simulink subsystem "PvtSubSys_PLAN_AP"  (R2020b)
settings: Solver=VariableStepAuto  StartTime=0.0  StopTime=10.0  RelTol=1e-3
undefined symbols (not defined in the file or in its folder): C_LongCtrl_0_Single, C_LongCtrl_0_Uint8, C_LongCtrl_Mph2Kph, magnitude, P_LongCtrl_accelTargAbsThrd, P_LongCtrl_AddVelAccelChange, P_LongCtrl_AddVelAccelThrd, P_LongCtrl_AddVelDistDesThrd, P_LongCtrl_AddVelEnable, P_LongCtrl_AddVelRefMsThrd, P_LongCtrl_ALaLowerChar, P_LongCtrl_ALaUpperCharEco, P_LongCtrl_ALaUpperCharNormal, P_LongCtrl_ALaUpperCharSport, P_LongCtrl_ALCAccLimitByDangerXAxis, P_LongCtrl_ALCAccLimitByDangerYAxis, P_LongCtrl_ALvAcceleLowerChar, P_LongCtrl_ALvAcceleUpperCharEco, P_LongCtrl_ALvAcceleUpperCharNormal, P_LongCtrl_ALvAcceleUpperCharSport, P_LongCtrl_CCaccelCCNeg2PosJerk, P_LongCtrl_CCaccelCCPosJerk, P_LongCtrl_CCaccelLowerIsLaneChange, P_LongCtrl_CCaccelMaxLCActive, P_LongCtrl_CCaccelMinECOAL, P_LongCtrl_CCaccelMinFastDecel, P_LongCtrl_CCaccelMinNoFastDecel, P_LongCtrl_CCaccelMinNormAL, P_LongCtrl_CCaccelMinSportAL, P_LongCtrl_CCaccelUpperCC, P_LongCtrl_CCaccelUpperCCSafeStop, P_LongCtrl_CCaMinNegAcceleLowerBand, P_LongCtrl_CCaMinNegAcceleUpperBand, P_LongCtrl_CCaMinPosAcceleLowerBand, P_LongCtrl_CCaMinPosAcceleUpperBand, P_LongCtrl_CCbECO, P_LongCtrl_CCbNorm, P_LongCtrl_CCbSport, P_LongCtrl_CCcoefESPSpd2IPSpd1, P_LongCtrl_CCcoefESPSpd2IPSpd2, P_LongCtrl_CCdecelCCJerk, P_LongCtrl_CCdecelCCJerkNegVLCInternalAcc, P_LongCtrl_CCfacNegAcceleLowerBand, P_LongCtrl_CCfacNegAcceleUpperBand, P_LongCtrl_CCfacPosAcceleLowerBand, P_LongCtrl_CCfacPosAcceleUpperBand, P_LongCtrl_CCkECO, P_LongCtrl_CCkNorm, P_LongCtrl_CCkSport, P_LongCtrl_CCLCIncSetSpdAdd, P_LongCtrl_CCLCIncSetSpdAddCntStartValue, P_LongCtrl_CCResumeDelayDeltaVel, P_LongCtrl_CCtAcceleTimeNeg, P_LongCtrl_CCtAcceleTimeNegCorrXAxis, P_LongCtrl_CCtAcceleTimeNegCorrYAxis, P_LongCtrl_CCtAcceleTimePos, P_LongCtrl_CCtAcceleTimePosCorrXAxis, P_LongCtrl_CCtAcceleTimePosCorrYAxis, P_LongCtrl_CCtStepVelPlan, P_LongCtrl_CCtTotVelPlan ... (+150)
libraries: simulink x62, TrueDurationTime x1
(part 3 of 7)

== system PvtSubSys_PLAN_AP/AP/AP/CCCtrl/accelCCJerkSelect ==
  VlcInternalAccK1 : Inport
  Compare To Constant : simulink/Logic and Bit Operations/Compare To Constant  relop=<  const=0  OutDataTypeStr=boolean
  Compare To Constant1 : simulink/Logic and Bit Operations/Compare To Constant  relop=>  const=0  OutDataTypeStr=boolean
  P_LongCtrl_CCaccelCCNeg2PosJerk : Constant  Value=P_LongCtrl_CCaccelCCNeg2PosJerk  OutDataTypeStr=single
  P_LongCtrl_CCaccelCCPosJerk : Constant  Value=P_LongCtrl_CCaccelCCPosJerk  OutDataTypeStr=single
  P_LongCtrl_CCdecelCCJerk : Constant  Value=P_LongCtrl_CCdecelCCJerk  OutDataTypeStr=single
  P_LongCtrl_CCdecelCCJerkNegVLCInternalAcc : Constant  Value=P_LongCtrl_CCdecelCCJerkNegVLCInternalAcc  OutDataTypeStr=single
  Switch : Switch  Criteria=u2 > Threshold
  Switch1 : Switch  Criteria=u2 > Threshold
  accelCCJerk : Outport
  decelCCJerk : Outport  Port=2
  wires:
  P_LongCtrl_CCdecelCCJerk/1 -> Switch1/1
  P_LongCtrl_CCdecelCCJerkNegVLCInternalAcc/1 -> Switch1/3  "decelCCJerk"
  Compare To Constant1/1 -> Switch1/2
  Switch1/1 -> decelCCJerk/1  "decelCCJerk"
  Switch/1 -> accelCCJerk/1  "accelCCJerk"
  P_LongCtrl_CCaccelCCPosJerk/1 -> Switch/3
  Compare To Constant/1 -> Switch/2
  VlcInternalAccK1/1 -> Compare To Constant/1, Compare To Constant1/1  "VlcInternalAccK1"
  P_LongCtrl_CCaccelCCNeg2PosJerk/1 -> Switch/1

== system PvtSubSys_PLAN_AP/AP/AP/CCCtrl/accelJerkCalc ==
  accelCCLim : Inport
  VlcInternalAcc : Inport  Port=2
  accelCCJerk : Inport  Port=3
  decelCCJerk : Inport  Port=4
  tCycle : Inport  Port=5
  Add : Sum
  Add1 : Sum
  MinMax : MinMax  Inputs=2
  MinMax1 : MinMax  Function=max  Inputs=2
  Product : Product
  Product1 : Product
  VlcInternalAcc1 : InportShadow  Port=2
  acceleratejerk1 : Constant  Value=4  OutDataTypeStr=single
  deceleratejerk1 : Constant  Value=-4  OutDataTypeStr=single
  accelCCDes : Outport
  upperJerkCC : Outport  Port=2
  lowerJerkCC : Outport  Port=3
  wires:
  acceleratejerk1/1 -> upperJerkCC/1  "upperJerkCC"
  deceleratejerk1/1 -> lowerJerkCC/1  "lowerJerkCC"
  MinMax1/1 -> accelCCDes/1  "accelCCDes"
  Add1/1 -> MinMax1/2
  Product1/1 -> Add1/2
  VlcInternalAcc1/1 -> Add1/1  "VlcInternalAcc"
  decelCCJerk/1 -> Product1/1
  tCycle/1 -> Product/2, Product1/2
  MinMax/1 -> MinMax1/1
  Add/1 -> MinMax/2
  Product/1 -> Add/2
  accelCCJerk/1 -> Product/1
  VlcInternalAcc/1 -> Add/1  "VlcInternalAcc"
  accelCCLim/1 -> MinMax/1

== system PvtSubSys_PLAN_AP/AP/AP/CCCtrl/velPlanCC ==
  VlcInternalAccK1 : Inport  OutDataTypeStr=single
  accelCCLim : Inport  Port=2
  fastDecel : Inport  Port=3
  DrivingMode : Inport  Port=4
  velSubj : Inport  Port=5  OutDataTypeStr=single
  Chart : Stateflow chart  TreatAsAtomicUnit=on
  Constant : Constant  Value=P_LongCtrl_CCdecelCCJerkNegVLCInternalAcc
  Constant1 : Constant  Value=P_LongCtrl_CCdecelCCJerk
  Constant10 : Constant  Value=P_LongCtrl_CCaccelMinNormAL  OutDataTypeStr=single
  Constant11 : Constant  Value=P_LongCtrl_CCbNorm  OutDataTypeStr=single
  Constant12 : Constant  Value=P_LongCtrl_CCkECO  OutDataTypeStr=single
  Constant13 : Constant  Value=P_LongCtrl_CCbSport  OutDataTypeStr=single
  Constant14 : Constant  Value=P_LongCtrl_CCkNorm  OutDataTypeStr=single
  Constant15 : Constant  Value=P_LongCtrl_CCbECO  OutDataTypeStr=single
  Constant16 : Constant  Value=P_LongCtrl_CCkSport  OutDataTypeStr=single
  Constant2 : Constant  Value=P_LongCtrl_CCaccelMinNoFastDecel
  Constant3 : Constant  Value=P_LongCtrl_CCaccelMinFastDecel
  Constant4 : Constant  Value=P_LongCtrl_CCtTotVelPlan  OutDataTypeStr=single
  Constant5 : Constant  Value=P_LongCtrl_CCtStepVelPlan  OutDataTypeStr=single
  Constant6 : Constant  Value=P_LongCtrl_CCaccelCCNeg2PosJerk  OutDataTypeStr=single
  Constant7 : Constant  Value=P_LongCtrl_CCaccelCCPosJerk  OutDataTypeStr=single
  Constant8 : Constant  Value=P_LongCtrl_CCaccelMinECOAL  OutDataTypeStr=single
  Constant9 : Constant  Value=P_LongCtrl_CCaccelMinSportAL  OutDataTypeStr=single
  velSubjPlanCC2ALC : Outport
  wires:
  DrivingMode/1 -> Chart/1(drivingMode)  "DrivingMode"
  velSubj/1 -> Chart/2(velSubj)  "velSubj"
  fastDecel/1 -> Chart/3(fastDecel)  "fastDecel"
  accelCCLim/1 -> Chart/4(accelCCLim)  "accelCCLim"
  VlcInternalAccK1/1 -> Chart/5(VLCInternalAccK1)  "VlcInternalAcc"
  Constant/1 -> Chart/6(P_LongCtrl_CCdecelCCJerkNegVLCInternalAcc)
  Constant1/1 -> Chart/7(P_LongCtrl_CCdecelCCJerk)
  Constant2/1 -> Chart/8(P_LongCtrl_CCaccelMinNoFastDecel)
  Constant3/1 -> Chart/9(P_LongCtrl_CCaccelMinFastDecel)
  Constant4/1 -> Chart/10(P_LongCtrl_CCtTotVelPlan)
  Constant5/1 -> Chart/11(P_LongCtrl_CCtStepVelPlan)
  Constant6/1 -> Chart/12(P_LongCtrl_CCaccelCCNeg2PosJerk)
  Constant7/1 -> Chart/13(P_LongCtrl_CCaccelCCPosJerk)
  Constant8/1 -> Chart/14(P_LongCtrl_CCaccelMinECOAL)
  Constant9/1 -> Chart/15(P_LongCtrl_CCaccelMinSportAL)
  Constant10/1 -> Chart/16(P_LongCtrl_CCaccelMinNormAL)
  Constant11/1 -> Chart/17(P_LongCtrl_CCbNorm)
  Constant14/1 -> Chart/18(P_LongCtrl_CCkNorm)
  Constant15/1 -> Chart/19(P_LongCtrl_CCbECO)
  Constant12/1 -> Chart/20(P_LongCtrl_CCkECO)
  Constant13/1 -> Chart/21(P_LongCtrl_CCbSport)
  Constant16/1 -> Chart/22(P_LongCtrl_CCkSport)
  Chart/1(velSubjPlanCC2ALC) -> velSubjPlanCC2ALC/1

== system PvtSubSys_PLAN_AP/AP/AP/FollowCtrl/AccelSupression ==
  accelFollow : Inport
  accelSubjPlanOpt : Inport  Port=2
  accelTargAbsEnable : Inport  Port=3
  velSubj : Inport  Port=4
  velTargRel : Inport  Port=5
  IDP0 : Inport  Port=6
  distTargRel : Inport  Port=7
  dangerLevel : Inport  Port=8
  laneChangeEnable : Inport  Port=9
  1-D Lookup Table : Lookup_n-D  NumberOfTableDimensions=1  BreakpointsForDimension1=P_LongCtrl_ALCAccLimitByDangerXAxis  Table=P_LongCtrl_ALCAccLimitByDangerYAxis  InternalRulePriority=Speed  RndMeth=Simplest  InputSameDT=on
  AccelSupression : Stateflow chart  TreatAsAtomicUnit=on
      settings: PortSchema="{\"entries\":[{\"content\":{\"sides\":[{\"content\":{\"connectorIds\":[\"In10\",\"In1\",\"In2\",\"In3\",\"In4\",\"In5\",\"In6\",\"In7\",\"In8\",\"In9\"]},\"type\":\"ConnectorPlacement.EquallySpacedRectSide\",\"uuid\":\"9300e1f1-bb95-41d4-adae-c883a64c9aa1\"},{\"content\":{\"connectorIds\":[\"Out1\",\"Out2\",\"Out3\"],\"side\":\"RIGHT\"},\"type\":\"ConnectorPlacement.EquallySpacedRectSide\",\"uuid\":\"008efea5-f081-441f-b580-11e25a33f47d\"},{\"content\":{\"connectorIds\":[],\"side\":\"TOP\"},\"type\":\"ConnectorPlacement.EquallySpacedRectSide\",\"uuid\":\"fa3bfdb5-3624-441a-b6df-0080d7c49dd2\"},{\"content\":{\"connectorIds\":[],\"side\":\"HIDDEN\"},\"type\":\"ConnectorPlacement.EquallySpacedRectSide\",\"uuid\":\"07e1617e-6ebd-494d-b9df-12fef96acb1d\"}]},\"type\":\"ConnectorPlacement.EquallySpacedConnector\",\"uuid\":\"901f3200-aee3-4515-88aa-e0e7a99820ae\"}],\"packageUris\":[\"http://schema.mathworks.com/mf0/Connector/R2020b\"],\"version\":\"1.0\"}"
  Constant : Constant  Value=P_LongCtrl_DangerLevelEnterThrd  OutDataTypeStr=single
  Constant2 : Constant  Value=P_LongCtrl_FollowaccelMinAccelSupressionEnter
  Constant3 : Constant  Value=P_LongCtrl_FollowaccelMinAccelSupressionExit
  Constant4 : Constant  Value=P_LongCtrl_DangerLevelExitThrd  OutDataTypeStr=single
  DecelJudge : MATLAB Function  TreatAsAtomicUnit=on
  MinMax : MinMax  Function=max  Inputs=2
  Signal Copy : SignalConversion  OverrideOpt=off
  Signal Copy1 : SignalConversion  OverrideOpt=off
  Switch : Switch  Criteria=u2 > Threshold
  Terminator : Terminator
  Terminator1 : Terminator
  accelFollowAfterLaneChangeSupress : Outport
  tStartDecel : Outport  Port=2
  wires:
  Signal Copy/1 -> AccelSupression/4(laneChangeEnable)  "LongCtrl_laneChangeEnable"
  Signal Copy1/1 -> AccelSupression/10(dangerLevel)  "LongCtrl_dangerLevel"
  dangerLevel/1 -> Signal Copy1/1, 1-D Lookup Table/1
  [accelFollow] -> MinMax/2
  MinMax/1 -> Switch/1
  Constant/1 -> AccelSupression/8(P_LongCtrl_DangerLevelEnterThrd)
  Constant4/1 -> AccelSupression/9(P_LongCtrl_DangerLevelExitThrd)
  accelTargAbsEnable/1 -> AccelSupression/2(accelTargAbsEnable)
  velSubj/1 -> AccelSupression/3(velSubj)
  velTargRel/1 -> AccelSupression/1(velTargRel)
  laneChangeEnable/1 -> Signal Copy/1
  accelSubjPlanOpt/1 -> DecelJudge/1(accelSubjPlanOpt)  "accelSubjPlanOpt"
  AccelSupression/1(accelSupressionEnable) -> Switch/2  "LongCtrl_accelSupressionEnable"
  1-D Lookup Table/1 -> MinMax/1  "LongCtrl_AccelSupreReq"
  accelFollow/1 -> Switch/3, [accelFollow]
  Switch/1 -> accelFollowAfterLaneChangeSupress/1  "LongCtrl_accelFollowAfterLaneChangeSupress"
  DecelJudge/1(tStartDecel) -> tStartDecel/1  "LongCtrl_tStartDecel"
  IDP0/1 -> DecelJudge/2(IDP0)  "IDP0"
  AccelSupression/2(distAccelSupressionMinEnter) -> Terminator/1  "LongCtrl_distAccelSupressionEnter"
  distTargRel/1 -> AccelSupression/5(distTargRel)
  Constant2/1 -> AccelSupression/6(P_LongCtrl_FollowaccelMinAccelSupressionEnter)
  Constant3/1 -> AccelSupression/7(P_LongCtrl_FollowaccelMinAccelSupressionExit)
  AccelSupression/3(distAccelSupressionMinExit) -> Terminator1/1  "LongCtrl_distAccelSupressionExit"

== system PvtSubSys_PLAN_AP/AP/AP/FollowCtrl/AccelTargAbsEnableJudge ==
  accelTargAbsFilt : Inport
  distTargRel : Inport  Port=2
  tCycle : Inport  Port=3
  IDP0 : Inport  Port=4  OutDataTypeStr=uint8
  AccelTargAbsEnableJudge : Stateflow chart  TreatAsAtomicUnit=on
  P_LongCtrl_FollowaccelTargAbsEnableNegJerk : Constant  Value=P_LongCtrl_FollowaccelTargAbsEnableNegJerk  OutDataTypeStr=single
  P_LongCtrl_FollowaccelTargAbsEnableNegMax : Constant  Value=P_LongCtrl_FollowaccelTargAbsEnableNegMax  OutDataTypeStr=single
  P_LongCtrl_FollowaccelTargAbsEnablePosJerk : Constant  Value=P_LongCtrl_FollowaccelTargAbsEnablePosJerk  OutDataTypeStr=single
  P_LongCtrl_FollowaccelTargAbsEnableRangeMax : Constant  Value=P_LongCtrl_FollowaccelTargAbsEnableRangeMax  OutDataTypeStr=single
  P_LongCtrl_FollowaccelTargAbsExitNegMin : Constant  Value=P_LongCtrl_FollowaccelTargAbsExitNegMin  OutDataTypeStr=single
  P_LongCtrl_FollowdistTargRelEnableAccelTargAbsThres : Constant  Value=P_LongCtrl_FollowdistTargRelEnableAccelTargAbsThres  OutDataTypeStr=single
  Tapped Delay : simulink/Discrete/Tapped Delay  vinit=0.0  samptime=-1  NumDelays=1  DelayOrder=Newest  includeCurrent=on
  accelTargAbsEnable : Outport
  wires:
  distTargRel/1 -> AccelTargAbsEnableJudge/2(distTargRel)
  tCycle/1 -> AccelTargAbsEnableJudge/4(tCycle)
  P_LongCtrl_FollowaccelTargAbsExitNegMin/1 -> AccelTargAbsEnableJudge/7(C_accelTargAbsExitNegMin)
  P_LongCtrl_FollowaccelTargAbsEnableRangeMax/1 -> AccelTargAbsEnableJudge/10(C_accelTargAbsEnableRangeMax)
  P_LongCtrl_FollowaccelTargAbsEnablePosJerk/1 -> AccelTargAbsEnableJudge/8(C_accelTargAbsEnablePosJerk)
  P_LongCtrl_FollowaccelTargAbsEnableNegMax/1 -> AccelTargAbsEnableJudge/5(C_accelTargAbsEnableNegMax)
  accelTargAbsFilt/1 -> AccelTargAbsEnableJudge/3(accelTargAbsFilt)
  P_LongCtrl_FollowdistTargRelEnableAccelTargAbsThres/1 -> AccelTargAbsEnableJudge/9(C_distTargRelEnableAccelTargAbsThres)
  P_LongCtrl_FollowaccelTargAbsEnableNegJerk/1 -> AccelTargAbsEnableJudge/6(C_accelTargAbsEnableNegJerk)
  AccelTargAbsEnableJudge/1(accelTargAbs) -> accelTargAbsEnable/1
  IDP0/1 -> Tapped Delay/1  "IDP0"
  Tapped Delay/1 -> AccelTargAbsEnableJudge/1(IDP0)

== system PvtSubSys_PLAN_AP/AP/AP/FollowCtrl/AccelTargFilter ==
  IDP0 : Inport  OutDataTypeStr=uint8
  IDP2 : Inport  Port=2  OutDataTypeStr=uint8
  IDP3 : Inport  Port=3  OutDataTypeStr=uint8
  accelTargAbsP0 : Inport  Port=4
  accelTargAbsP2 : Inport  Port=5
  accelTargAbsP3 : Inport  Port=6
  Tapped Delay : simulink/Discrete/Tapped Delay  vinit=0.0  samptime=-1  NumDelays=1  DelayOrder=Newest  includeCurrent=on
  Tapped Delay1 : simulink/Discrete/Tapped Delay  vinit=0.0  samptime=-1  NumDelays=1  DelayOrder=Newest  includeCurrent=on
  Tapped Delay2 : simulink/Discrete/Tapped Delay  vinit=0.0  samptime=-1  NumDelays=1  DelayOrder=Newest  includeCurrent=on
  accelTargAbsFilter : Stateflow chart  TreatAsAtomicUnit=on
  accelTargAbsFilt : Outport
  wires:
  Tapped Delay2/1 -> accelTargAbsFilter/3(IDP3)
  Tapped Delay1/1 -> accelTargAbsFilter/2(IDP2)
  Tapped Delay/1 -> accelTargAbsFilter/1(IDP0)
  accelTargAbsP3/1 -> accelTargAbsFilter/6(accelTargAbsP3)
  accelTargAbsP2/1 -> accelTargAbsFilter/5(accelTargAbsP2)
  IDP3/1 -> Tapped Delay2/1
  IDP2/1 -> Tapped Delay1/1
  IDP0/1 -> Tapped Delay/1  "IDP0"
  accelTargAbsP0/1 -> accelTargAbsFilter/4(accelTargAbsP0)
  accelTargAbsFilter/1(accelTargAbsFiltP0) -> accelTargAbsFilt/1  "accelTargAbsFilt"

== system PvtSubSys_PLAN_AP/AP/AP/FollowCtrl/DecelToStopCtrl ==
  accelFollow : Inport
  distDesCur : Inport  Port=2
  velTargAbs : Inport  Port=3
  accelTargAbsFilt : Inport  Port=4
  distTargRel : Inport  Port=5
  velSubj : Inport  Port=6
  ACCModeSts : Inport  Port=7  OutDataTypeStr=uint8
  DrvOFF_Req : Inport  Port=8
  axvRoadSlopeMs2 : Inport  Port=9
  ObjMovingStateP0 : Inport  Port=10
  DecelToStopCtrl : Subsystem
  accelFollowAfterDecelToStop : Outport
  ForceStop : Outport  Port=2
  wires:
  ObjMovingStateP0/1 -> DecelToStopCtrl/10(ObjMovingStateP0)
  DrvOFF_Req/1 -> DecelToStopCtrl/8(DrvOFF_Req)
  velTargAbs/1 -> DecelToStopCtrl/6(velTargAbs)
  ACCModeSts/1 -> DecelToStopCtrl/7(ACCModeSts)
  distDesCur/1 -> DecelToStopCtrl/5(distDesCur)
  DecelToStopCtrl/1(FollowAccel) -> accelFollowAfterDecelToStop/1  "LongCtrl_accelFollowAfterDecelToStop"
  accelTargAbsFilt/1 -> DecelToStopCtrl/2(accelTargAbs)
  distTargRel/1 -> DecelToStopCtrl/3(distTargRel)
  velSubj/1 -> DecelToStopCtrl/4(velSubj)
  accelFollow/1 -> DecelToStopCtrl/1(FollowAccelMPC)  "accelFollwBeforeDecelToStop"
  axvRoadSlopeMs2/1 -> DecelToStopCtrl/9(axvRoadSlopeMs2)
  DecelToStopCtrl/2(ForceStop) -> ForceStop/1  "LongCtrl_ForceStop"

== system PvtSubSys_PLAN_AP/AP/AP/FollowCtrl/DistDesCalc ==
  velTargAbsPlanTerminate : Inport
  timeGap : Inport  Port=2
  distTargRel : Inport  Port=3
  velTargRel : Inport  Port=4
  velSubj : Inport  Port=5
  1-D Lookup Table : Lookup_n-D  NumberOfTableDimensions=1  BreakpointsForDimension1=P_LongCtrl_FollowdistDesCompensionXAxis  Table=P_LongCtrl_FollowdistDesCompensionYAxis  ExtrapMethod=Clip  InternalRulePriority=Speed  RndMeth=Simplest  InputSameDT=on
  Constant36 : Constant  Value=P_LongCtrl_FollowDistDesCompensionVelRelThresMin  OutDataTypeStr=single
  Constant37 : Constant  Value=P_LongCtrl_FollowDistDesCompensionVelRelThresMax  OutDataTypeStr=single
  DesireDistance1 : Lookup_n-D  BreakpointsForDimension1=[1,2,3,4]  BreakpointsForDimension2=P_LongCtrl_FollowdistDesX2Axis  BreakpointsForDimension1DataTypeStr=single  BreakpointsForDimension2DataTypeStr=single  Table=P_LongCtrl_FollowdistDesYAxis  TableDataTypeStr=single  ExtrapMethod=Clip  OutDataTypeStr=single  RndMeth=Simplest
      settings: InputPortMap=u0,u1
  DesireDistance2 : Lookup_n-D  BreakpointsForDimension1=[1,2,3,4]  BreakpointsForDimension2=P_LongCtrl_FollowdistDesX2Axis  BreakpointsForDimension1DataTypeStr=single  BreakpointsForDimension2DataTypeStr=single  Table=P_LongCtrl_FollowdistDesYAxis  TableDataTypeStr=single  ExtrapMethod=Clip  OutDataTypeStr=single  RndMeth=Simplest
      settings: InputPortMap=u0,u1
  DesireDistance3 : Lookup_n-D  BreakpointsForDimension1=[1,2,3,4]  BreakpointsForDimension2=P_LongCtrl_FollowdistDesX2Axis  BreakpointsForDimension1DataTypeStr=single  BreakpointsForDimension2DataTypeStr=single  Table=P_LongCtrl_FollowdistDesYAxis  TableDataTypeStr=single  ExtrapMethod=Clip  OutDataTypeStr=single  RndMeth=Simplest
      settings: InputPortMap=u0,u1
  Gain9 : Gain  Gain=3.6
  Lookup Table Dynamic : simulink/Lookup Tables/Lookup Table Dynamic  LookUpMeth=Interpolation-Use End Values  OutDataType=fixdt('single')  OutScaling=[]  OutputDataTypeScalingMode=Specify via dialog  OutDataTypeStr=single  DoSatur=off
  Matrix Concatenate1 : Concatenate
  Matrix Concatenate2 : Concatenate
  Min : MinMax  Inputs=2
  Subtract1 : Sum
  Subtract2 : Sum  Inputs=-+
  Subtract5 : Sum
  distDesPlanCorr : Outport
  distDesCur : Outport  Port=2
  wires:
  Subtract2/1 -> Matrix Concatenate2/1
  DesireDistance2/1 -> distDesCur/1
  [timeGap] -> DesireDistance2/1
  velSubj/1 -> Subtract1/2, DesireDistance2/2, 1-D Lookup Table/1
  [distTargRel] -> Subtract2/1
  DesireDistance1/1 -> Subtract2/2
  Subtract1/1 -> DesireDistance1/2
  [timeGap] -> DesireDistance1/1
  Min/1 -> distDesPlanCorr/1
  Subtract5/1 -> Min/2
  distTargRel/1 -> [distTargRel], Subtract5/1
  Lookup Table Dynamic/1 -> Subtract5/2
  Matrix Concatenate2/1 -> Lookup Table Dynamic/3
  Constant36/1 -> Matrix Concatenate1/1
  Gain9/1 -> Lookup Table Dynamic/1
  1-D Lookup Table/1 -> Matrix Concatenate2/2
  Constant37/1 -> Matrix Concatenate1/2
  Matrix Concatenate1/1 -> Lookup Table Dynamic/2
  velTargRel/1 -> Subtract1/1, Gain9/1
  velTargAbsPlanTerminate/1 -> DesireDistance3/2
  DesireDistance3/1 -> Min/1  "LongCtrl_distDesPlan"
  timeGap/1 -> [timeGap], DesireDistance3/1

== system PvtSubSys_PLAN_AP/AP/AP/FollowCtrl/DistRelPlanTerminateCalc ==
  accelTargAbsEnable : Inport
  velTargAbs : Inport  Port=2
  velTargAbsPlanTerminate : Inport  Port=3
  distDesPlanCorr : Inport  Port=4
  distTargRel : Inport  Port=5
  velSubj : Inport  Port=6
  1-D Lookup Table : Lookup_n-D  NumberOfTableDimensions=1  BreakpointsForDimension1=[0 2]  Table=[0 2]  ExtrapMethod=Clip  InternalRulePriority=Speed  RndMeth=Simplest  InputSameDT=on
  DistRelPlanTerminateCalc2 : MATLAB Function  TreatAsAtomicUnit=on
  distRelPlanTerminate : Outport
  tTargStop : Outport  Port=2
  distTargPlan : Outport  Port=3
  wires:
  DistRelPlanTerminateCalc2/3(distTargPlan) -> distTargPlan/1
  DistRelPlanTerminateCalc2/2(tTargStop) -> tTargStop/1
  1-D Lookup Table/1 -> DistRelPlanTerminateCalc2/6(DterminateMin)
  velSubj/1 -> DistRelPlanTerminateCalc2/7(velSubj), 1-D Lookup Table/1
  velTargAbs/1 -> DistRelPlanTerminateCalc2/4(vf)
  DistRelPlanTerminateCalc2/1(Dterminate) -> distRelPlanTerminate/1  "distRelPlanTerminate"
  velTargAbsPlanTerminate/1 -> DistRelPlanTerminateCalc2/3(velTargAbsPlanTerminate)
  distDesPlanCorr/1 -> DistRelPlanTerminateCalc2/2(distDesPlanCorr)
  distTargRel/1 -> DistRelPlanTerminateCalc2/1(R)
  accelTargAbsEnable/1 -> DistRelPlanTerminateCalc2/5(af)

== system PvtSubSys_PLAN_AP/AP/AP/FollowCtrl/FollowBandJerkCalc ==
  Gap : Inport
  accelFollow : Inport  Port=2
  PlauCheckEnable : Inport  Port=3
  ttc : Inport  Port=4
  ForceStop : Inport  Port=5
  VlcInternalAccK1 : Inport  Port=6
  distTargRel : Inport  Port=7
  velSubj : Inport  Port=8
  ACCModeSts : Inport  Port=9  OutDataTypeStr=uint8
  tCycle : Inport  Port=10
  velTargRel : Inport  Port=11
  IDP0 : Inport  Port=12
  axvRoadSlopeMs2 : Inport  Port=13
  accelTargAbsFilt : Inport  Port=14
  AccelFollowAfterJerk : Subsystem
  AccelFollowJerkCalc : Subsystem
  DecelFollowJerkCalc : Subsystem
  LP : Subsystem
  Subsystem : Subsystem
  Terminator : Terminator
  upperBandFollow : Outport
  lowerBandFollow : Outport  Port=2
  " upperJerkFollow" : Outport  Port=3
  lowerJerkFollow : Outport  Port=4
  accelFollowAfterJerk : Outport  Port=5
  wires:
  accelTargAbsFilt/1 -> DecelFollowJerkCalc/10(accelTargAbsFilt)
  PlauCheckEnable/1 -> Terminator/1
  ttc/1 -> DecelFollowJerkCalc/7(ttc)
  velTargRel/1 -> DecelFollowJerkCalc/6(velTargRel)
  Gap/1 -> DecelFollowJerkCalc/5(Gap)
  tCycle/1 -> AccelFollowAfterJerk/3(tCycle), DecelFollowJerkCalc/1(tCycle)
  distTargRel/1 -> DecelFollowJerkCalc/2(distTargRel)
  velSubj/1 -> [velSubj], DecelFollowJerkCalc/3(velSubj)
  ACCModeSts/1 -> DecelFollowJerkCalc/4(ACCModeSts)
  VlcInternalAccK1/1 -> AccelFollowAfterJerk/2(VlcInternalAccK1), AccelFollowJerkCalc/1(VlcInternalAccK1), DecelFollowJerkCalc/11(VlcInternalAccK1)
  DecelFollowJerkCalc/1(decelFollowJerk) -> lowerJerkFollow/1, AccelFollowAfterJerk/4(lowerJerkFollow)  "LongCtrl_lowerJerkFollow"
  AccelFollowJerkCalc/1(accelFollowJerk) -> " upperJerkFollow"/1, AccelFollowAfterJerk/5(" upperJerkFollow")  "LongCtrl_upperJerkFollow"
  LP/1(accelFollowFilt) -> AccelFollowJerkCalc/2(FollowAccele), Subsystem/1(accelFollowFilt), AccelFollowAfterJerk/1(accelFollow)  "accelFollow"
  AccelFollowAfterJerk/1(accelFollowAfterJerk) -> accelFollowAfterJerk/1
  Subsystem/1(upperBandFollow) -> upperBandFollow/1
  Subsystem/2(lowerBandFollow) -> lowerBandFollow/1
  accelFollow/1 -> LP/1(accelFollow)  "accelFollow"
  ForceStop/1 -> DecelFollowJerkCalc/8(ForceStop)
  IDP0/1 -> LP/2(IDP0)
  axvRoadSlopeMs2/1 -> DecelFollowJerkCalc/9(axvRoadSlopeMs2)
  [velSubj] -> AccelFollowJerkCalc/3(velSubj)

== system PvtSubSys_PLAN_AP/AP/AP/FollowCtrl/PlausibilityCheck ==
  FollowAcceleK1 : Inport
  accelSubjPlan : Inport  Port=2
  num : Inport  Port=3
  velTargAbs : Inport  Port=4
  distRelPlanTerminate : Inport  Port=5
  velSubj : Inport  Port=6
  IDP0 : Inport  Port=7
  distTargRel : Inport  Port=8
  ACCMode : Inport  Port=9
  velTargRel : Inport  Port=10
  accelTargAbsEnable : Inport  Port=11
  distDesCur : Inport  Port=12
  Bus Creator : BusCreator  Inputs=12
  Bus Selector : BusSelector  OutputSignals=accelSubjPlan,velSubj,velTargAbs,distRelPlanTerminate,num,IDP0,FollowAcceleK1,distTargRel
  Bus Selector1 : BusSelector  OutputSignals=velTargAbs,distTargRel,ACCMode
  Bus Selector2 : BusSelector  OutputSignals=velTargRel,accelTargAbsEnable,distDesCur,velSubj,distTargRel
  PlausibilityCheck : MATLAB Function  TreatAsAtomicUnit=on
  StandstillOverride : Stateflow chart  TreatAsAtomicUnit=on
  StandstillOverrideAccelLimit : Subsystem
  Subsystem : Subsystem
  Tapped Delay : simulink/Discrete/Tapped Delay  vinit=0.0  samptime=-1  NumDelays=1  DelayOrder=Newest  includeCurrent=on
  PlauCheckEnable : Outport
  followAcceleStandstillOverride : Outport  Port=2
  wires:
  Bus Selector1/3 -> StandstillOverride/4(ACCMode)  "<ACCMode>"
  Bus Selector1/1 -> StandstillOverride/2(velTargAbs)  "<velTargAbs>"
  Bus Selector1/2 -> StandstillOverride/3(distTargRel)  "<distTargRel>"
  StandstillOverrideAccelLimit/1(followAcceleStandstillOverride) -> followAcceleStandstillOverride/1  "followAcceleStandstillOverride"
  StandstillOverride/2(coefStandstillOverride) -> StandstillOverrideAccelLimit/3(coefStandstillOverride)  "LongCtrl_coefStandstillOverride"
  ACCMode/1 -> Bus Creator/9  "ACCMode"
  Bus Selector/8 -> PlausibilityCheck/8(distTargRel)  "<distTargRel>"
  Bus Selector/7 -> PlausibilityCheck/7(FollowAcceleK1)  "<FollowAcceleK1>"
  Bus Selector/6 -> Tapped Delay/1  "<IDP0>"
  Bus Selector/5 -> PlausibilityCheck/5(num)  "<num>"
  Bus Selector/4 -> PlausibilityCheck/4(distRelPlanTerminate)  "<distRelPlanTerminate>"
  Bus Selector/3 -> PlausibilityCheck/3(velTargAbs)  "<velTargAbs>"
  Bus Selector/2 -> PlausibilityCheck/2(velSubj)  "<velSubj>"
  Bus Selector/1 -> PlausibilityCheck/1(FollowAccele)  "<accelSubjPlan>"
  Bus Creator/1 -> Bus Selector2/1, Bus Selector1/1, Bus Selector/1
  distTargRel/1 -> Bus Creator/8  "distTargRel"
  FollowAcceleK1/1 -> Bus Creator/7  "FollowAcceleK1"
  IDP0/1 -> Bus Creator/6  "IDP0"
  num/1 -> Bus Creator/5  "num"
  distRelPlanTerminate/1 -> Bus Creator/4  "distRelPlanTerminate"
  velTargAbs/1 -> Bus Creator/3  "velTargAbs"
  velSubj/1 -> Bus Creator/2  "velSubj"
  accelSubjPlan/1 -> Bus Creator/1  "accelSubjPlan"
  PlausibilityCheck/2(PlauCheckEnable) -> PlauCheckEnable/1
  Tapped Delay/1 -> PlausibilityCheck/6(IDP0)
  PlausibilityCheck/1(FollowAccele_Plau) -> StandstillOverride/1(FollowAccele_Plau), StandstillOverrideAccelLimit/1(followAccel_Plau)  "LongCtrl_followAccel_Plau"
  StandstillOverride/1(standstillOverrideCondition) -> StandstillOverrideAccelLimit/2(standstillOverrideCondition)  "LongCtrl_standstillOverrideCondition"
  velTargRel/1 -> Bus Creator/10  "velTargRel"
  accelTargAbsEnable/1 -> Bus Creator/11  "accelTargAbsEnable"
  distDesCur/1 -> Bus Creator/12  "distDesCur"
  Bus Selector2/1 -> Subsystem/1(velTargRel)  "<velTargRel>"
  Bus Selector2/2 -> Subsystem/2(accelTargAbsEnable)  "<accelTargAbsEnable>"
  Bus Selector2/3 -> Subsystem/3(distDesCur)  "<distDesCur>"
  Bus Selector2/4 -> Subsystem/4(velSubj)  "<velSubj>"
  Bus Selector2/5 -> Subsystem/5(distTargRel)  "<distTargRel>"
  Subsystem/1(quickDecel) -> StandstillOverrideAccelLimit/4(quickDecel)  "LongCtrl_quickDecel"

== system PvtSubSys_PLAN_AP/AP/AP/FollowCtrl/SlopeStartupAssist ==
  accelFollowAfterLaneChangeSupress : Inport
  axvRoadSlopeMs2 : Inport  Port=2
  velSubj : Inport  Port=3
  velTargRel : Inport  Port=4
  distTargRel : Inport  Port=5
  ACCModeSts : Inport  Port=6  OutDataTypeStr=uint8
  tCycle : Inport  Port=7
  distDesCur : Inport  Port=8
  velTargAbs : Inport  Port=9
  1-D Lookup Table : Lookup_n-D  NumberOfTableDimensions=1  BreakpointsForDimension1=P_LongCtrl_FollowAccelAddSlopeAssistXAxis  Table=P_LongCtrl_FollowAccelAddSlopeAssistYAxis  ExtrapMethod=Clip  InternalRulePriority=Speed  RndMeth=Simplest  InputSameDT=on
  Add : Sum
  Chart : Stateflow chart  TreatAsAtomicUnit=on
  Chart1 : Stateflow chart  TreatAsAtomicUnit=on
  Compare To Constant : simulink/Logic and Bit Operations/Compare To Constant  relop=<=  const=2  OutDataTypeStr=boolean
  Compare To Constant1 : simulink/Logic and Bit Operations/Compare To Constant  relop=>  const=0.8  OutDataTypeStr=boolean
  Compare To Constant2 : simulink/Logic and Bit Operations/Compare To Constant  relop=<  const=0.5  OutDataTypeStr=boolean
  Compare To Constant3 : simulink/Logic and Bit Operations/Compare To Constant  relop=>  const=0.15  OutDataTypeStr=boolean
  Constant : Constant  Value=P_LongCtrl_FollowAccelSlopeAssistStep  OutDataTypeStr=single
  Logical Operator : Logic  Inputs=4  AllPortsSameDT=off  OutDataTypeStr=boolean
  Product : Product
  accelFollowSlopeAssist : Outport
  wires:
  accelFollowAfterLaneChangeSupress/1 -> Chart1/2(accelFollowAfterLaneChangeSupress), Add/1, Compare To Constant3/1, Compare To Constant2/1
  axvRoadSlopeMs2/1 -> 1-D Lookup Table/1, Compare To Constant1/1  "axvRoadSlopeMs2"
  velSubj/1 -> Chart1/1(velSubj), Compare To Constant/1  "velSubj"
  Compare To Constant2/1 -> Logical Operator/1
  Compare To Constant3/1 -> Logical Operator/2
  Compare To Constant1/1 -> Logical Operator/4
  Compare To Constant/1 -> Logical Operator/3
  Logical Operator/1 -> Chart/1(slopeStartupAssist)  "LongCtrl_slopeStartupAssist"
  1-D Lookup Table/1 -> Chart/2(accelSlopeAssistMax)
  Constant/1 -> Chart/3(accelSlopeAssistStep)
  Add/1 -> Product/1
  Chart/1(accelSlopeAssist) -> Add/2  "LongCtrl_accelFollowSlopeAssist"
  velTargAbs/1 -> Chart1/3(velTargAbs)
  distDesCur/1 -> Chart1/4(distDesCur)
  distTargRel/1 -> Chart1/5(distTargRel)
  velTargRel/1 -> Chart1/6(velTargRel)
  ACCModeSts/1 -> Chart1/7(ACCModeSts)
  tCycle/1 -> Chart1/8(tCycle)
  Chart1/1(coefVelDist2Accel) -> Product/2  "LongCtrl_coefVelDist2AccelStartUp"
  Product/1 -> accelFollowSlopeAssist/1

== system PvtSubSys_PLAN_AP/AP/AP/FollowCtrl/TTC ==
  velTargRel : Inport
  distTargRel : Inport  Port=2
  Constant : Constant  Value=0.01  OutDataTypeStr=single
  Gain : Gain  Gain=-1
  MinMax : MinMax  Function=max  Inputs=2
  Product1 : Product  Inputs=*/
  ttc : Outport
  wires:
  Gain/1 -> MinMax/1
  Constant/1 -> MinMax/2
  Product1/1 -> ttc/1
  MinMax/1 -> Product1/2
  velTargRel/1 -> Gain/1
  distTargRel/1 -> Product1/1

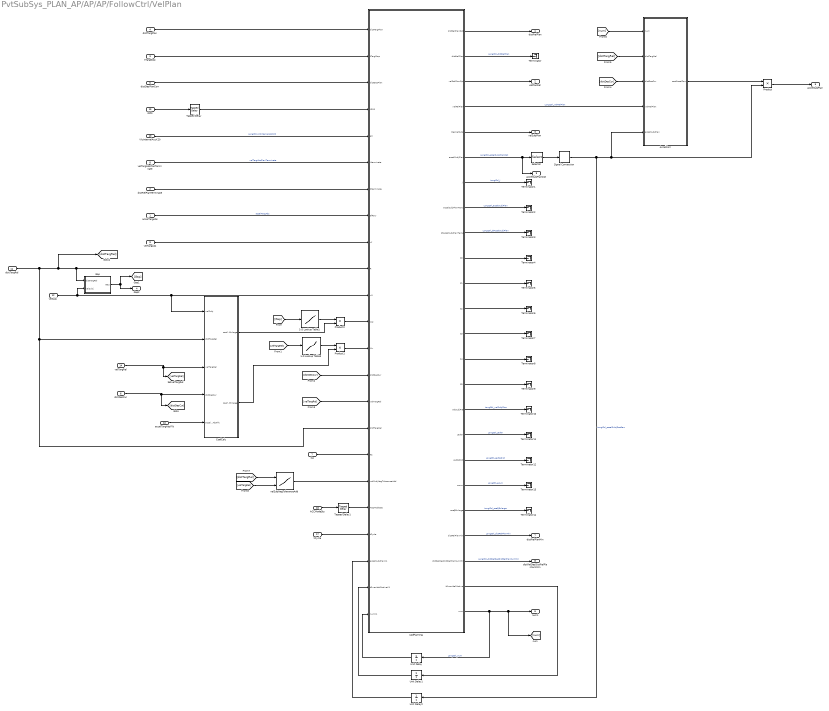
== system PvtSubSys_PLAN_AP/AP/AP/FollowCtrl/VelPlan ==
  accelTargAbs : Inport
  distRelPlanTerminate : Inport  Port=2
  tTargStop : Inport  Port=3
  distTargPlan : Inport  Port=4
  distDesPlanCorr : Inport  Port=5
  distDesCur : Inport  Port=6
  ttc : Inport  Port=7
  velTargAbsPlanTerminate : Inport  Port=8
  velTargAbs : Inport  Port=9
  accelTargAbsFilt : Inport  Port=10
  distTargRel : Inport  Port=11
  velSubj : Inport  Port=12
  VlcInternalAccK20 : Inport  Port=13
  velTargRel : Inport  Port=14
  IDP0 : Inport  Port=15  OutDataTypeStr=uint8
  ACCModeSts : Inport  Port=16  OutDataTypeStr=uint8
  tCycle : Inport  Port=17
  1-D Lookup Table1 : Lookup_n-D  NumberOfTableDimensions=1  BreakpointsForDimension1=P_LongCtrl_FollowWdCoefXAxis  Table=P_LongCtrl_FollowWdCoefYAxis  ExtrapMethod=Clip  InternalRulePriority=Speed  RndMeth=Simplest  InputSameDT=on
  1-D Lookup Table3 : Lookup_n-D  NumberOfTableDimensions=1  BreakpointsForDimension1=P_LongCtrl_FollowWvCoefXAxis  Table=P_LongCtrl_FollowWvCoefYAxis  ExtrapMethod=Clip  InternalRulePriority=Speed  RndMeth=Simplest  InputSameDT=on
  AccelCorr : MATLAB Function  TreatAsAtomicUnit=on
  CoefCalc : MATLAB Function  TreatAsAtomicUnit=on
  Gap : Subsystem
  Product : Product
  Product1 : Product
  Product2 : Product
  Selector : Selector  InputPortWidth=40  IndexOptions=Index vector (dialog)  Indices=1  OutputSizes=1
  Signal Conversion : SignalConversion  OverrideOpt=off
  Tapped Delay : simulink/Discrete/Tapped Delay  vinit=0.0  samptime=-1  NumDelays=1  DelayOrder=Newest  includeCurrent=on
  Tapped Delay1 : simulink/Discrete/Tapped Delay  vinit=0.0  samptime=-1  NumDelays=1  DelayOrder=Newest  includeCurrent=on
  Terminator{,1..14} (15 alike) : Terminator
  Unit Delay : UnitDelay  InitialCondition=2  SampleTime=-1  HasFrameUpgradeWarning=on
  Unit Delay1 : UnitDelay  SampleTime=-1  HasFrameUpgradeWarning=on
  Unit Delay2 : UnitDelay  SampleTime=-1  HasFrameUpgradeWarning=on
  spdPlanning : MATLAB Function  TreatAsAtomicUnit=on
  velSubjNegToleranceAdd : Lookup_n-D  BreakpointsForDimension1=P_LongCtrl_FollowVelSubjNegToleranceAddX1Axis  BreakpointsForDimension2=P_LongCtrl_FollowVelSubjNegToleranceAddX2Axis  Table=P_LongCtrl_FollowVelSubjNegToleranceAddYAxis  ExtrapMethod=Clip  InternalRulePriority=Speed  RndMeth=Simplest  InputSameDT=on
      settings: InputPortMap=u0,u1
  distRelPlan : Outport  OutDataTypeStr=single
  velPlanRel : Outport  Port=2  OutDataTypeStr=single
  velSubjPlan : Outport  Port=3  OutDataTypeStr=single
  Gap2 : Outport  Port=4  OutDataTypeStr=single
  accelSubjPlan : Outport  Port=5  OutDataTypeStr=single
  num1 : Outport  Port=6  OutDataTypeStr=single
  distRelPlanMin : Outport  Port=7  OutDataTypeStr=single
  distRelDesDistRelPlanNumMin : Outport  Port=8  OutDataTypeStr=single
  accelSubjPlanOpt : Outport  Port=9
  wires:
  ACCModeSts/1 -> Tapped Delay1/1
  velSubjNegToleranceAdd/1 -> spdPlanning/18(velSubjNegToleranceAdd)
  [velTargRel] -> velSubjNegToleranceAdd/2
  [distTargRel] -> velSubjNegToleranceAdd/1
  tCycle/1 -> spdPlanning/20(tCycle)
  Tapped Delay1/1 -> spdPlanning/19(ACCModeSts)
  Unit Delay1/1 -> spdPlanning/22(tOverride2ActiveK1)
  spdPlanning/23(tOverride2Active) -> Unit Delay1/1
  Signal Conversion/1 -> AccelCorr/5(accelSubjPlan), Product/2, Unit Delay2/1  "LongCtrl_accelSubjDesRaw"
  CoefCalc/2(coefVelEnlarge) -> Product1/2
  ttc/1 -> spdPlanning/17(ttc)
  spdPlanning/22(distRelDesDistRelPlanNumMin) -> distRelDesDistRelPlanNumMin/1  "LongCtrl_distRelDesDistRelPlanNumMin"
  spdPlanning/21(distRelPlanMin) -> distRelPlanMin/1  "LongCtrl_distRelPlanMin"
  Tapped Delay/1 -> spdPlanning/4(IDP0)
  [num] -> AccelCorr/1(num)
  Product/1 -> accelSubjPlan/1
  Selector/1 -> Signal Conversion/1
  AccelCorr/1(coefAccelCorr) -> Product/1
  spdPlanning/4(velRelPlan) -> AccelCorr/4(velRelPlan)  "LongCtrl_velRelPlan"
  [distTargRel] -> AccelCorr/2(distTargRel)
  [distDesCur] -> AccelCorr/3(distDesCur)
  CoefCalc/1(coefDistEnlarge) -> Product2/2
  Product1/1 -> spdPlanning/13(Wv)
  [velTargRel] -> spdPlanning/15(velTargRel)
  spdPlanning/20(coefJEnlarge) -> Terminator14/1  "LongCtrl_coefJEnlarge"
  Gap/1(Gap) -> [Gap], Gap2/1
  Unit Delay2/1 -> spdPlanning/21(accelSubjPlanK1)
  [distDesCur] -> spdPlanning/14(distDesCur)
  accelTargAbsFilt/1 -> CoefCalc/5(accelTargAbsFilt)
  VlcInternalAccK20/1 -> spdPlanning/5(a0)  "LongCtrl_VlcInternalAccK20"
  Product2/1 -> spdPlanning/12(Wd)
  [velTargRel] -> 1-D Lookup Table3/1
  1-D Lookup Table3/1 -> Product1/1
  [Gap] -> 1-D Lookup Table1/1
  distTargPlan/1 -> spdPlanning/1(distTargPlan)
  tTargStop/1 -> spdPlanning/2(tTargStop)
  spdPlanning/18(JadtADist) -> Terminator12/1  "LongCtrl_JadtADist"
  1-D Lookup Table1/1 -> Product2/1
  distDesPlanCorr/1 -> spdPlanning/3(distDesPlan)
  spdPlanning/2(distRelPlan) -> Terminator/1  "LongCtrl_distRelPlan"
  spdPlanning/19(asum) -> Terminator13/1  "LongCtrl_asum"
  spdPlanning/17(JadtA) -> Terminator11/1  "LongCtrl_JadtA"
  IDP0/1 -> Tapped Delay/1
  Unit Delay/1 -> spdPlanning/23(numK1)
  spdPlanning/16(velSubjPre) -> Terminator10/1  "LongCtrl_velSubjPlan"
  spdPlanning/15(C5) -> Terminator9/1
  spdPlanning/14(C4) -> Terminator8/1
  spdPlanning/13(C3) -> Terminator7/1
  spdPlanning/12(C2) -> Terminator6/1
  spdPlanning/11(C1) -> Terminator5/1
  spdPlanning/10(C0) -> Terminator4/1
  distDesCur/1 -> [distDesCur], CoefCalc/4(distDesCur)
  velTargRel/1 -> CoefCalc/3(velTargRel), [velTargRel]
  spdPlanning/9(dtAccelSubjPlanTemp) -> Terminator3/1  "LongCtrl_dtAccelSubjPlan"
  spdPlanning/8(accelSubjPlanTemp) -> Terminator2/1  "LongCtrl_accelSubjPlan"
  spdPlanning/7(J) -> Terminator1/1  "LongCtrl_J"
  spdPlanning/6(accelSubjPlan) -> Selector/1, accelSubjPlanOpt/1  "LongCtrl_accelSubjPlanOpt"
  spdPlanning/24(num) -> num1/1, [num], Unit Delay/1  "LongCtrl_num"
  velSubj/1 -> spdPlanning/11(v0), CoefCalc/1(velSubj), Gap/2(velSubj)
  spdPlanning/1(distRelPlanOpt) -> distRelPlan/1
  spdPlanning/5(DesVelSubj) -> velSubjPlan/1
  velTargAbs/1 -> spdPlanning/9(vf)
  spdPlanning/3(velRelPlanOpt) -> velPlanRel/1
  velTargAbsPlanTerminate/1 -> spdPlanning/6(Vterminate)  "velTargAbsPlanTerminate"
  distTargRel/1 -> spdPlanning/10(R), Gap/1(distTargRel), [distTargRel], spdPlanning/16(distTargRel), CoefCalc/2(distTargRel)
  accelTargAbs/1 -> spdPlanning/8(afRaw)  "accelTargAbs"
  distRelPlanTerminate/1 -> spdPlanning/7(Dterminate)

== system PvtSubSys_PLAN_AP/AP/AP/FollowCtrl/VelTargPlanTerminateCalc ==
  accelTargAbsEnable : Inport
  velTargRel : Inport  Port=2
  velSubj : Inport  Port=3
  Constant2 : Constant  Value=0  OutDataTypeStr=single
  MinMax : MinMax  Function=max  Inputs=2
  Subtract3 : Sum
  VelTarAbsTerminateCalc : MATLAB Function  TreatAsAtomicUnit=on
  velTargAbs : Outport
  velTargAbsPlanTerminate : Outport  Port=2
  wires:
  Subtract3/1 -> MinMax/1
  Constant2/1 -> MinMax/2
  velSubj/1 -> Subtract3/2
  MinMax/1 -> VelTarAbsTerminateCalc/1(vf), velTargAbs/1
  VelTarAbsTerminateCalc/1(vterminate) -> velTargAbsPlanTerminate/1  "LongCtrl_velTargAbsPlanTerminate"
  velTargRel/1 -> Subtract3/1
  accelTargAbsEnable/1 -> VelTarAbsTerminateCalc/2(af)

== system PvtSubSys_PLAN_AP/AP/AP/IC/AccelArbIC ==
  note: IC_state=1,道路曲率限速；
      | IC_state=2,行驶轨迹曲率限速
  accelMap : Inport
  accelCurvature : Inport  Port=2
  accelKap : Inport  Port=3
  MATLAB Function : MATLAB Function  TreatAsAtomicUnit=on
  accelIC : Outport
  IC_state : Outport  Port=2
  wires:
  MATLAB Function/2(IC_state) -> IC_state/1
  MATLAB Function/1(accelIC) -> accelIC/1
  accelKap/1 -> MATLAB Function/3(accelKap)  "accelKap"
  accelCurvature/1 -> MATLAB Function/2(accelCurvature)  "accelCurvature"
  accelMap/1 -> MATLAB Function/1(accelMap)

== system PvtSubSys_PLAN_AP/AP/AP/IC/AccelBandIC ==
  accelIC : Inport
  P_LongCtrl_ICdeltaAccelLowerBand : Constant  Value=P_LongCtrl_ICdeltaAccelLowerBand  OutDataTypeStr=single
  P_LongCtrl_ICdeltaAccelUpperBand : Constant  Value=P_LongCtrl_ICdeltaAccelUpperBand  OutDataTypeStr=single
  Sum1 : Sum  Inputs=|++
  Sum2 : Sum  Inputs=+-|  OutDataTypeStr=single
  upperBandIC : Outport
  lowerBandIC : Outport  Port=2
  wires:
  Sum2/1 -> lowerBandIC/1
  Sum1/1 -> upperBandIC/1
  P_LongCtrl_ICdeltaAccelLowerBand/1 -> Sum2/2
  P_LongCtrl_ICdeltaAccelUpperBand/1 -> Sum1/1
  accelIC/1 -> Sum1/2, Sum2/1

== system PvtSubSys_PLAN_AP/AP/AP/IC/AccelCurvature ==
  curvatureForCurveDecel : Inport
  velSubj : Inport  Port=2
  1-D Lookup Table2 : Lookup_n-D  NumberOfTableDimensions=1  BreakpointsForDimension1=P_LongCtrl_ICCurvatureLimitSpdXAxis  Table=P_LongCtrl_ICCurvatureLimitSpdYAxis  ExtrapMethod=Clip  InternalRulePriority=Speed  RndMeth=Simplest  InputSameDT=on
  Add : Sum  Inputs=+-
  Constant2 : Constant  Value=P_LongCtrl_ICtDecel
  Constant7 : Constant  Value=0.0001  OutDataTypeStr=single
  Divide : Product  Inputs=*/
  Gain2 : Gain  Gain=1/3.6
  MinMax5 : MinMax  Function=max  Inputs=2
  accelCurvature : Outport
  wires:
  Add/1 -> Divide/1
  Gain2/1 -> Add/1
  curvatureForCurveDecel/1 -> MinMax5/1
  MinMax5/1 -> 1-D Lookup Table2/1
  Constant7/1 -> MinMax5/2
  velSubj/1 -> Add/2
  Divide/1 -> accelCurvature/1  "LongCtrl_accelCurvature"
  Constant2/1 -> Divide/2
  1-D Lookup Table2/1 -> Gain2/1

== system PvtSubSys_PLAN_AP/AP/AP/IC/AccelKap ==
  velSubj : Inport
  kap : Inport  Port=2
  1-D Lookup Table : Lookup_n-D  NumberOfTableDimensions=1  BreakpointsForDimension1=[0 4 8]  Table=[10 10 10]  ExtrapMethod=Clip  InternalRulePriority=Speed  RndMeth=Simplest  InputSameDT=on
  1-D Lookup Table1 : Lookup_n-D  NumberOfTableDimensions=1  BreakpointsForDimension1=P_LongCtrl_ICKapLimitAccelXAxis  Table=P_LongCtrl_ICKapLimitAccelYAxis  ExtrapMethod=Clip  InternalRulePriority=Speed  RndMeth=Simplest  InputSameDT=on
  1-D Lookup Table3 : Lookup_n-D  NumberOfTableDimensions=1  BreakpointsForDimension1=P_LongCtrl_ICKapLimitSpdXAxis  Table=P_LongCtrl_ICKapLimitSpdYAxis  ExtrapMethod=Clip  InternalRulePriority=Speed  RndMeth=Simplest  InputSameDT=on
  Abs : Abs
  Add1 : Sum  Inputs=+-
  Constant1 : Constant  Value=0.0001  OutDataTypeStr=single
  Constant2 : Constant  Value=P_LongCtrl_ICtDecel
  Divide1 : Product  Inputs=*/
  Gain : Gain  Gain=1.2
  Gain4 : Gain  Gain=1/3.6
  LP : Subsystem
  MinMax1 : MinMax  Function=max  Inputs=2  OutDataTypeStr=single
  MinMax3 : MinMax  Function=max  Inputs=2
  MinMax4 : MinMax  Inputs=2  OutDataTypeStr=single
  accelKap : Outport
  wires:
  1-D Lookup Table1/1 -> MinMax1/2  "LongCtrl_accelKapStartupRaw"
  1-D Lookup Table/1 -> MinMax1/1
  Gain4/1 -> Add1/1
  Gain/1 -> Abs/1
  Abs/1 -> MinMax3/1
  Add1/1 -> Divide1/1
  LP/1(Out1) -> Gain/1
  Constant1/1 -> MinMax3/2
  1-D Lookup Table3/1 -> Gain4/1
  MinMax4/1 -> accelKap/1  "LongCtrl_accelKap"
  Divide1/1 -> MinMax4/1  "LongCtrl_accelKapRun"
  kap/1 -> LP/1(In1)
  MinMax3/1 -> 1-D Lookup Table3/1, 1-D Lookup Table1/1  "LongCtrl_kapFilt"
  MinMax1/1 -> MinMax4/2  "LongCtrl_accelKapStartup"
  velSubj/1 -> 1-D Lookup Table/1, Add1/2
  Constant2/1 -> Divide1/2

== system PvtSubSys_PLAN_AP/AP/AP/IC/CurvatureOfMapCalc ==
  velSubj : Inport
  i_road_curvature : Inport  Port=2
  i_road_curvature_far : Inport  Port=3
  i_road_curvature_far_distance : Inport  Port=4
  i_road_curvature_value_matrix : Inport  Port=5
  i_road_curvature_distance_matrix : Inport  Port=6
  i_road_curvature_matrix_size : Inport  Port=7
  Abs : Abs
  Chart : Stateflow chart  TreatAsAtomicUnit=on
  LP : Subsystem  TreatAsAtomicUnit=on
  Math Function : Math  Operator=transpose  SaturateOnIntegerOverflow=on
  Math Function1 : Math  Operator=transpose  SaturateOnIntegerOverflow=on
  Signal Conversion{,1..5} (6 alike) : SignalConversion  OverrideOpt=off
  Terminator{,1..4} (5 alike) : Terminator
  accelDesCurvatureMap : Outport
  wires:
  i_road_curvature_far_distance/1 -> Signal Conversion4/1
  i_road_curvature_far/1 -> Signal Conversion3/1
  i_road_curvature/1 -> Signal Conversion/1
  Signal Conversion5/1 -> Chart/3(LongCtrl_IC_EHRV2_CurMatrixSize)  "LongCtrl_IC_EHRV2_CurMatrixSize"
  Signal Conversion3/1 -> Terminator/1  "LongCtrl_IC_EHRV2_CurFar"
  Signal Conversion4/1 -> Terminator1/1  "LongCtrl_IC_EHRV2_CurFarDis"
  Signal Conversion/1 -> Terminator2/1  "LongCtrl_IC_EHRV2_Cur"
  Signal Conversion2/1 -> Math Function1/1  "LongCtrl_IC_EHRV2_CurDisMatrix"
  Signal Conversion1/1 -> LP/1(LongCtrl_IC_EHRV2_CurMatrix)  "LongCtrl_IC_EHRV2_CurMatrix"
  LP/1(LongCtrl_IC_EHRV2_CurMatrixLP) -> Math Function/1
  Math Function/1 -> Abs/1
  Math Function1/1 -> Chart/2(LongCtrl_IC_EHRV2_CurDisMatrix)
  i_road_curvature_value_matrix/1 -> Signal Conversion1/1
  i_road_curvature_distance_matrix/1 -> Signal Conversion2/1
  i_road_curvature_matrix_size/1 -> Signal Conversion5/1
  velSubj/1 -> Chart/4(velSubj)
  Chart/1(accelICCurvatureMapMatrix) -> Terminator3/1  "LongCtrl_accelICCurvatureMapMatrix"
  Chart/2(distDesCurvatureMap) -> Terminator4/1  "LongCtrl_distDesCurvatureMap"
  Chart/3(accelDesCurvatureMap) -> accelDesCurvatureMap/1  "LongCtrl_accelDesCurvatureMap"
  Abs/1 -> Chart/1(LongCtrl_IC_EHRV2_CurMatrixLP)

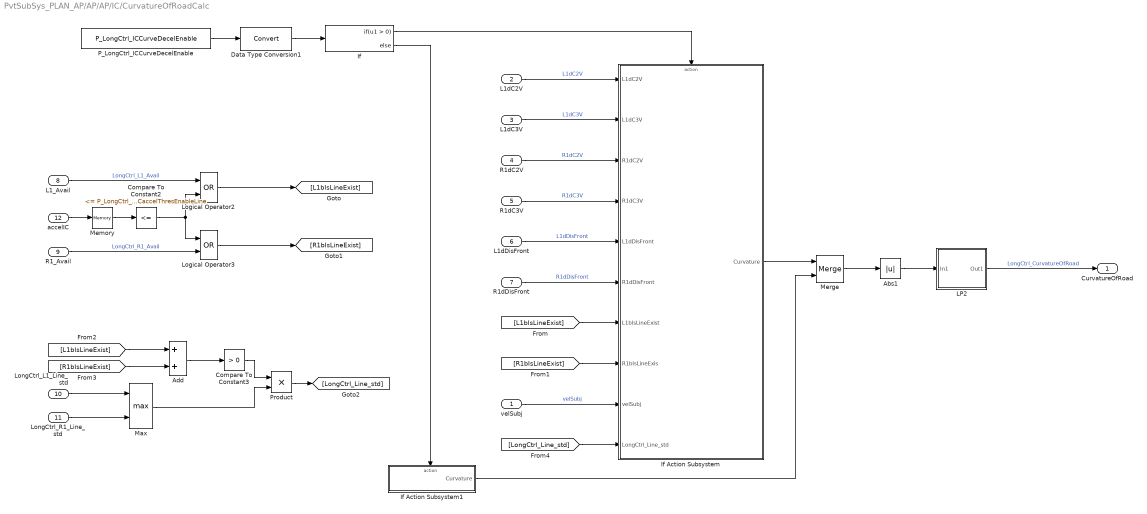
== system PvtSubSys_PLAN_AP/AP/AP/IC/CurvatureOfRoadCalc ==
  velSubj : Inport
  L1dC2V : Inport  Port=2
  L1dC3V : Inport  Port=3
  R1dC2V : Inport  Port=4
  R1dC3V : Inport  Port=5
  L1dDisFront : Inport  Port=6
  R1dDisFront : Inport  Port=7
  L1_Avail : Inport  Port=8
  R1_Avail : Inport  Port=9
  LongCtrl_L1_Line_std : Inport  Port=10
  LongCtrl_R1_Line_std : Inport  Port=11
  accelIC : Inport  Port=12
  Abs1 : Abs
  Add : Sum
  Compare To Constant2 : simulink/Logic and Bit Operations/Compare To Constant  relop=<=  const=P_LongCtrl_ICaccelThresEnableLine  OutDataTypeStr=boolean
  Compare To Constant3 : simulink/Logic and Bit Operations/Compare To Constant  relop=>  const=0  OutDataTypeStr=boolean
  Data Type Conversion1 : DataTypeConversion
  If : If
  If Action Subsystem : Subsystem  TreatAsAtomicUnit=on
  If Action Subsystem1 : Subsystem  TreatAsAtomicUnit=on
  LP2 : Subsystem
  Logical Operator2 : Logic  Operator=OR  AllPortsSameDT=off  OutDataTypeStr=boolean
  Logical Operator3 : Logic  Operator=OR  AllPortsSameDT=off  OutDataTypeStr=boolean
  Max : MinMax  Function=max  Inputs=2
  Memory : Memory  InheritSampleTime=on
  Merge : Merge
  P_LongCtrl_ICCurveDecelEnable : Constant  Value=P_LongCtrl_ICCurveDecelEnable
  Product : Product
  CurvatureOfRoad : Outport
  wires:
  [R1bIsLineExist] -> If Action Subsystem/8(R1bIsLineExis)
  [L1bIsLineExist] -> If Action Subsystem/7(L1bIsLineExist)
  Logical Operator2/1 -> [L1bIsLineExist]
  R1dC3V/1 -> If Action Subsystem/4(R1dC3V)  "R1dC3V"
  R1dDisFront/1 -> If Action Subsystem/6(R1dDisFront)  "R1dDisFront"
  L1dC2V/1 -> If Action Subsystem/1(L1dC2V)  "L1dC2V"
  velSubj/1 -> If Action Subsystem/9(velSubj)  "velSubj"
  L1dC3V/1 -> If Action Subsystem/2(L1dC3V)  "L1dC3V"
  L1dDisFront/1 -> If Action Subsystem/5(L1dDisFront)  "L1dDisFront"
  R1dC2V/1 -> If Action Subsystem/3(R1dC2V)  "R1dC2V"
  If Action Subsystem1/1(Curvature) -> Merge/2
  Data Type Conversion1/1 -> If/1
  P_LongCtrl_ICCurveDecelEnable/1 -> Data Type Conversion1/1
  LP2/1(Out1) -> CurvatureOfRoad/1  "LongCtrl_CurvatureOfRoad"
  Merge/1 -> Abs1/1
  If Action Subsystem/1(Curvature) -> Merge/1
  If/1 -> If Action Subsystem/Action
  Abs1/1 -> LP2/1(In1)
  If/2 -> If Action Subsystem1/Action
  accelIC/1 -> Memory/1
  Memory/1 -> Compare To Constant2/1
  L1_Avail/1 -> Logical Operator2/1  "LongCtrl_L1_Avail"
  Logical Operator3/1 -> [R1bIsLineExist]
  R1_Avail/1 -> Logical Operator3/2  "LongCtrl_R1_Avail"
  Compare To Constant2/1 -> Logical Operator3/1, Logical Operator2/2
  [L1bIsLineExist] -> Add/1
  [R1bIsLineExist] -> Add/2
  Add/1 -> Compare To Constant3/1
  LongCtrl_L1_Line_std/1 -> Max/1
  LongCtrl_R1_Line_std/1 -> Max/2
  Max/1 -> Product/2
  Compare To Constant3/1 -> Product/1
  Product/1 -> [LongCtrl_Line_std]
  [LongCtrl_Line_std] -> If Action Subsystem/10(LongCtrl_Line_std)

== system PvtSubSys_PLAN_AP/AP/AP/IC/JerkIC ==
  accelIC : Inport
  IC_state : Inport  Port=2
  VlcInternalAcc : Inport  Port=3
  1-D Lookup Table : Lookup_n-D  NumberOfTableDimensions=1  BreakpointsForDimension1=P_LongCtrl_ICupperJerkICCharXAxis  Table=P_LongCtrl_ICupperJerkICCharYAxis  ExtrapMethod=Clip  InternalRulePriority=Speed  RndMeth=Simplest  InputSameDT=on
  1-D Lookup Table1 : Lookup_n-D  NumberOfTableDimensions=1  BreakpointsForDimension1=P_LongCtrl_IClowerJerkICCharXAxis  Table=P_LongCtrl_IClowerJerkICCharYAxis  ExtrapMethod=Clip  InternalRulePriority=Speed  RndMeth=Simplest  InputSameDT=on
  Constant : Constant  Value=P_LongCtrl_IClowerJerkPosVLCInternalAccMin
  Constant1 : Constant  Value=P_LongCtrl_IClowerJerkPosVLCInternalAccMax
  Constant2 : Constant  Value=P_LongCtrl_ICUpperJerkNegVLCInternalAcc
  Constant3 : Constant  Value=P_LongCtrl_ICUpperJerkNegVLCInternalAcc
  Min : MinMax  Inputs=2
  Multiport Switch : MultiPortSwitch  Inputs=2
  Saturation : Saturate  UpperLimit=10  LowerLimit=P_LongCtrl_ICKapUpperJerkMin
  Switch : Switch  Criteria=u2 > Threshold
  Switch1 : Switch  Criteria=u2 > Threshold
  Switch2 : Switch  Criteria=u2 > Threshold
  upperJerkIC : Outport
  LowerJerkIC : Outport  Port=2
  wires:
  Saturation/1 -> Switch2/1
  Multiport Switch/1 -> upperJerkIC/1
  IC_state/1 -> Multiport Switch/1
  1-D Lookup Table/1 -> Switch1/1, Saturation/1
  accelIC/1 -> 1-D Lookup Table/1, 1-D Lookup Table1/1
  Min/1 -> LowerJerkIC/1
  VlcInternalAcc/1 -> [VlcInternalAcc], Switch/2  "VlcInternalAcc"
  Constant/1 -> Switch/1
  Constant1/1 -> Switch/3
  1-D Lookup Table1/1 -> Min/1
  Switch/1 -> Min/2
  [VlcInternalAcc] -> Switch1/2
  Switch1/1 -> Multiport Switch/2
  [VlcInternalAcc] -> Switch2/2
  Switch2/1 -> Multiport Switch/3
  Constant2/1 -> Switch1/3
  Constant3/1 -> Switch2/3
